simulink model "classification_model"  (R2018b)
settings: Solver=daessc  StartTime=0.0  StopTime=1  RelTol=1e-3
libraries: powerlib x7, powerlib_meascontrol x2
CloseFcn:
  | % location = 200;
  | % fault = 1010;
  | % urrent = c(:,2:4);
  | % current(:,4) = fault;
  | % current(:,5) = location;
  | % voltage = v(:,2:4);
  | % logg = [voltage,current];
  | % data = xlsread('sdata');
  | % data = [data;logg];
  | % xlswrite('sdata',data);
settings Model: Creator=Edagotti Pavankumar  LastModifiedBy=dedeepya
settings SolverCC: ZeroCrossAlgorithm=Adaptive
settings DebuggingCC: IgnoredZcDiagnostic=none

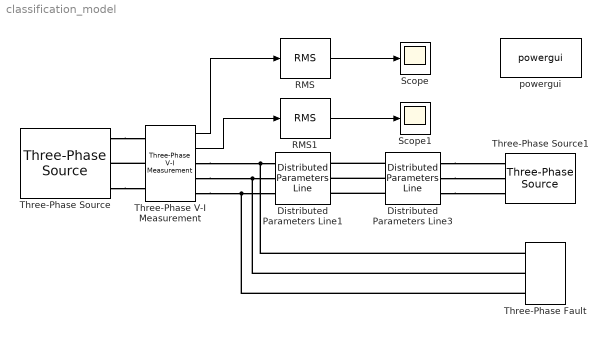
== system classification_model ==
  Distributed Parameters Line1 : powerlib/Elements/Distributed Parameters Line  Phases=3  Frequency=50  Resistance=[0.0238 0.3885]  Inductance=[0.0009509508 0.0032508989]  Capacitance=[12.74e-9 7.751e-9]  Length=50  x1=[7.20466777852578e-10 243580.547693811 243580.547693813;314.159265358979 314.159265358979 314.159265358979;-2.86994580460193 0.453303789111017 -1.11749253768387]  x2=[8.4479476656816e-10 243945.210549292 243945.210549294;314.159265358979 314.159265358979 314.159265358979;-3.08219944153453 0.453191852184442 -1.11760447461045]  x3=[4.98124015712591e-12 890.094635964552 890.094635964556;314.159265358979 314.159265358979 314.159265358979;1.34528005457524 0.398576748209828 -1.17221957858507]  x4=[4.11960733054362e-12 889.860414529128 889.860414529134;314.159265358979 314.159265358979 314.159265358979;-2.1072147617435 0.453192099220105 -1.11760422757479]  x5=0.000250986639952707  V1=[7.205e-10 2.436e+05 2.436e+05;314.2 314.2 314.2;-2.87 0.4533 -1.117]  V2=[8.448e-10 2.439e+05 2.439e+05;314.2 314.2 314.2;-3.082 0.4532 -1.118]  I1=[4.981e-12 890.1 890.1;314.2 314.2 314.2;1.345 0.3986 -1.172]  I2=[4.12e-12 889.9 889.9;314.2 314.2 314.2;-2.107 0.4532 -1.118]  nHarmo=1  Measurements=None
      settings: SourceProductName=Simscape Power Systems
  Distributed Parameters Line3 : powerlib/Elements/Distributed Parameters Line  Phases=3  Frequency=50  Resistance=[0.0238 0.3885]  Inductance=[0.0009509508 0.0032508989]  Capacitance=[12.74e-9 7.751e-9]  Length=50  x1=[8.4479476656816e-10 243945.210549292 243945.210549294;314.159265358979 314.159265358979 314.159265358979;-3.08219944153453 0.453191852184442 -1.11760447461045]  x2=[7.36275143029257e-10 243580.836046556 243580.836046558;314.159265358979 314.159265358979 314.159265358979;-2.89869187761561 0.453318294972105 -1.11747803182279]  x3=[3.52793946391785e-12 890.096596134685 890.096596134689;314.159265358979 314.159265358979 314.159265358979;-1.65758244652482 0.453191605214322 -1.11760472158057]  x4=[3.39338407563962e-12 889.859481632832 889.859481632843;314.159265358979 314.159265358979 314.159265358979;1.35121635438221 0.398577271582454 -1.17221905521245]  x5=0.000250986639952707  V1=[8.448e-10 2.439e+05 2.439e+05;314.2 314.2 314.2;-3.082 0.4532 -1.118]  V2=[7.363e-10 2.436e+05 2.436e+05;314.2 314.2 314.2;-2.899 0.4533 -1.117]  I1=[3.528e-12 890.1 890.1;314.2 314.2 314.2;-1.658 0.4532 -1.118]  I2=[3.393e-12 889.9 889.9;314.2 314.2 314.2;1.351 0.3986 -1.172]  nHarmo=1  Measurements=None
      settings: SourceProductName=Simscape Power Systems
  RMS : powerlib_meascontrol/Measurements/RMS  TrueRMS=on  Freq=50  RMSInit=0  Ts=0
  RMS1 : powerlib_meascontrol/Measurements/RMS  TrueRMS=on  Freq=50  RMSInit=0  Ts=0
  Scope : Scope
  Scope1 : Scope
  Three-Phase V-I Measurement : powerlib/Measurements/Three-Phase V-I Measurement  VoltageMeasurement=phase-to-ground  SetLabelV=off  LabelV=Vabc  Vpu=on  VpuLL=off  CurrentMeasurement=yes  SetLabelI=off  LabelI=Iabc  Ipu=on  Pbase=100e6  Vbase=220e3  OutputType=Complex  PhasorSimulation=off  PSBequivalent=0
  Three-Phase Fault : powerlib/Elements/Three-Phase Fault  InitialStates=0  FaultA=on  FaultB=on  FaultC=on  GroundFault=on  SwitchTimes=2  External=off  SwitchStatus=NaN  FaultResistance=0.001  GroundResistance=0.001  SnubberResistance=1e6  SnubberCapacitance=inf  Measurements=None
  Three-Phase Source : powerlib/Electrical Sources/Three-Phase Source  InternalConnection=Yg  VoltagePhases=off  Voltage=220e3  PhaseAngle=0  Voltage_phases=[25e3 25e3 25e3]/sqrt(3)  PhaseAngles_phases=[0 -120 +120]  Frequency=50  NonIdealSource=on  SpecifyImpedance=on  Resistance=0.8929  Inductance=16.58e-3  ShortCircuitLevel=100e6  BaseVoltage=220e3  XRratio=7  BusType=swing  Pref=10e3  Qref=0  Prefabc=[10e3, 10e3, 10e3]  Qrefabc=[0, 0, 0]  Qmin=-inf  Qmax=inf
  Three-Phase Source1 : powerlib/Electrical Sources/Three-Phase Source  InternalConnection=Yg  VoltagePhases=off  Voltage=220e3  PhaseAngle=0  Voltage_phases=[25e3 25e3 25e3]/sqrt(3)  PhaseAngles_phases=[0 -120 +120]  Frequency=50  NonIdealSource=on  SpecifyImpedance=on  Resistance=0.8929  Inductance=16.58e-3  ShortCircuitLevel=100e6  BaseVoltage=220e3  XRratio=7  BusType=swing  Pref=10e3  Qref=0  Prefabc=[10e3, 10e3, 10e3]  Qrefabc=[0, 0, 0]  Qmin=-inf  Qmax=inf
  powergui : powerlib/powergui  Priority=1  SimulationMode=Continuous  SampleTime=50e-10  frequency=60  Iterations=50  frequencyindice=50  Pbase=100e6  ErrMax=1e-4  UnitsV=kV  UnitsW=MW  buscounter=0  FunctionMessages=off  echomessages=off  EnableUseOfTLC=off  CurrentSourceSwitches=off  DisableSnubberDevices=off  DisableRonSwitches=off  DisableVfSwitches=off  DisplayEquations=off  SolverType=Tustin/Backward Euler (TBE)  Interpol=off  ExternalGateDelay=off  methode=off  Ts=100  x0status=blocks  SPID=off  SwTol=0  HookPort=off  RestoreLinks=warning  ResistiveCurrentMeasurement=off  Frange=[0:2:500]  Ylog=off  Xlog=on  ShowGrid=off  save=off  variable=ZData  structure=0  ZoomFFT=off  StartTime=0.0  cycles=1  DisplayStyle=1  fundamental=60  FreqAxis=off  MaxFrequency=1000  frequencyindicesteady=1  RmsSteady=2  display=off
  wires:
  Three-Phase V-I Measurement/1 -> RMS/1
  RMS/1 -> Scope/1
  RMS1/1 -> Scope1/1
  Three-Phase V-I Measurement/2 -> RMS1/1
  connections:
  Three-Phase V-I Measurement/LConn2 -- Three-Phase Source/RConn2
  Three-Phase Source/RConn1 -- Three-Phase V-I Measurement/LConn1
  Three-Phase Source/RConn3 -- Three-Phase V-I Measurement/LConn3
  Three-Phase V-I Measurement/RConn1 -- Three-Phase Fault/LConn1 -- Distributed Parameters Line1/LConn1
  Three-Phase V-I Measurement/RConn2 -- Three-Phase Fault/LConn2 -- Distributed Parameters Line1/LConn2
  Three-Phase V-I Measurement/RConn3 -- Three-Phase Fault/LConn3 -- Distributed Parameters Line1/LConn3
  Distributed Parameters Line3/RConn1 -- Three-Phase Source1/RConn1
  Distributed Parameters Line3/RConn2 -- Three-Phase Source1/RConn2
  Distributed Parameters Line3/RConn3 -- Three-Phase Source1/RConn3
  Distributed Parameters Line3/LConn1 -- Distributed Parameters Line1/RConn1
  Distributed Parameters Line3/LConn2 -- Distributed Parameters Line1/RConn2
  Distributed Parameters Line3/LConn3 -- Distributed Parameters Line1/RConn3
